simulink model "Task_No5"  (R2023b)
settings: Solver=FixedStepAuto  StartTime=0.0  StopTime=3600*24*7  FixedStep=1  RelTol=1e-3
InitFcn:
  | PARAMETERS;
StartFcn:
  | PARAMETERS;
undefined symbols (not defined in the file): Conv_C_to_K, P_CP_AIR, P_DENSITY_CO2, P_HEATER_AIR_FLOW, P_INIT_CO2, P_M_AIR, P_M_AIR_FLOW, R_WALL, R_WINDOW, RH_INIT_BDR, T_COOLER, T_HEATER, T_INIT_BDR, T_INIT_OUT, TBL_CO2, TBL_TEMP
libraries: fl_lib x32, nesl_utility x20, slpidlib x2
settings Model: Creator=Selim  LastModifiedBy=Selim

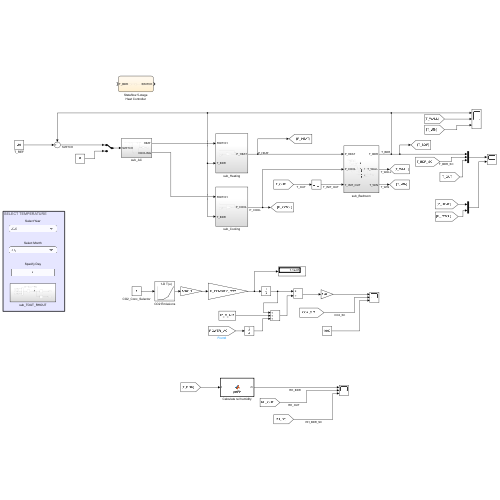
[thumbnail: Simulink's stored preview of the top-level diagram]
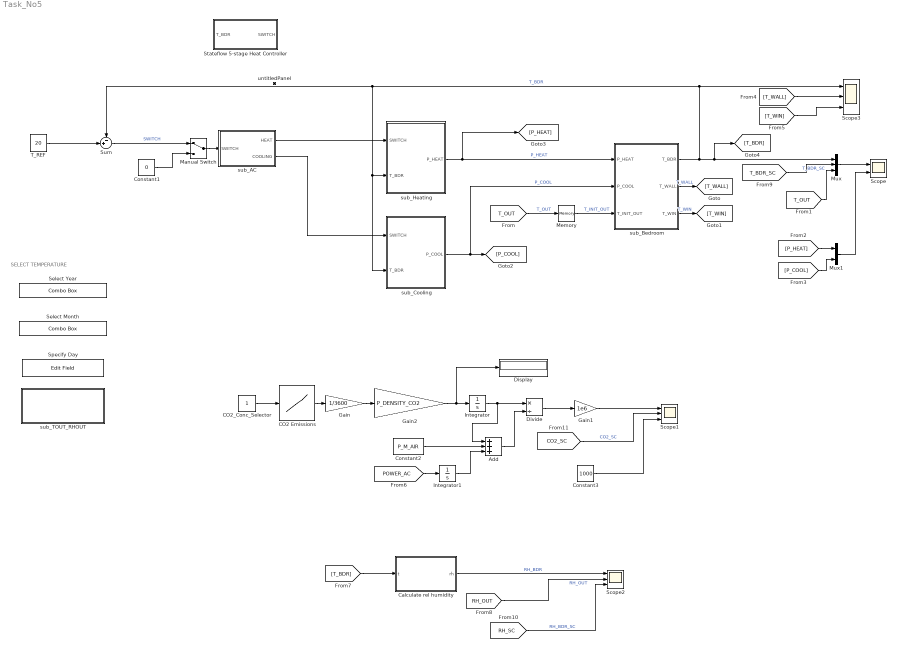
== system Task_No5 ==
  note: SELECT TEMPERATURE
  Add : Sum  Inputs=+++
  CO2 Emissions : Lookup_n-D  NumberOfTableDimensions=1  BreakpointsForDimension1=TBL_CO2.Activity_ID  Table=TBL_CO2.CO2_Emiss_cmh  InternalRulePriority=Speed  RndMeth=Simplest
  CO2_Conc_Selector : Constant
  Calculate rel humidity : MATLAB Function  TreatAsAtomicUnit=on
  Constant1 : Constant  Value=0
  Constant2 : Constant  Value=P_M_AIR
  Constant3 : Constant  Value=1000
  Display : Display
  Divide : Product  Inputs=*/
  Gain : Gain  Gain=1/3600
  Gain1 : Gain  Gain=1e6
  Gain2 : Gain  Gain=P_DENSITY_CO2
  Integrator : Integrator
  Integrator1 : Integrator
  Manual Switch : ManualSwitch
  Memory : Memory  InitialCondition=T_INIT_OUT
  Mux : Mux  Inputs=3
  Mux1 : Mux  Inputs=2
  Scope : Scope  NumInputPorts=2
  Scope1 : Scope  NumInputPorts=3
  Scope2 : Scope  NumInputPorts=3
  Scope3 : Scope  NumInputPorts=3
  Select Month : ComboBox  LabelPosition=Hide  SelectedLabel=July
      settings: Values={{'January', 'February', 'March', 'April', 'May', 'June', 'July', 'August', 'September', 'Oktober', 'November', 'December'}, [1 2 3 4 5 6 7 8 9 10 11 12]}
  Select Year : ComboBox  LabelPosition=Hide  SelectedLabel=2023
      settings: Values={{'2022', '2023'}, [2022 2023]}
  Specify Day : EditField  LabelPosition=Hide  ShowInitialText=on  Alignment=Center
  Stateflow 5-stage Heat Controller : Stateflow chart  TreatAsAtomicUnit=on
  Sum : Sum  Inputs=-+|
  T_REF : Constant  Value=20
  sub_AC : Subsystem
  sub_Bedroom : Subsystem
  sub_Cooling : Subsystem
  sub_Heating : Subsystem
  sub_TOUT_RHOUT : Subsystem
  untitledPanel : Subsystem  Tag=HiddenForWebPanel  IsWebBlockPanel=on
  wires:
  Memory/1 -> sub_Bedroom/3(T_INIT_OUT)  "T_INIT_OUT"
  sub_Bedroom/1(T_BDR) -> [T_BDR], Mux/1, Sum/1, sub_Cooling/2(T_BDR), sub_Heating/2(T_BDR), Scope3/1  "T_BDR"
  sub_Heating/1(P_HEAT) -> [P_HEAT], sub_Bedroom/1(P_HEAT)  "P_HEAT"
  [T_OUT] -> Memory/1  "T_OUT"
  [T_OUT] -> Mux/3
  Mux/1 -> Scope/1
  T_REF/1 -> Sum/2
  Mux1/1 -> Scope/2
  Sum/1 -> Manual Switch/1  "SWITCH"
  sub_AC/1(HEAT) -> sub_Heating/1(SWITCH)
  Manual Switch/1 -> sub_AC/1(SWITCH)
  Constant1/1 -> Manual Switch/2
  sub_Cooling/1(P_COOL) -> [P_COOL], sub_Bedroom/2(P_COOL)  "P_COOL"
  sub_Bedroom/2(T_WALL) -> [T_WALL]  "T_WALL"
  sub_Bedroom/3(T_WIN) -> [T_WIN]  "T_WIN"
  [P_HEAT] -> Mux1/1
  [P_COOL] -> Mux1/2
  [T_WALL] -> Scope3/2
  [T_WIN] -> Scope3/3
  CO2_Conc_Selector/1 -> CO2 Emissions/1
  CO2 Emissions/1 -> Gain/1
  Integrator/1 -> Add/1, Divide/1
  Add/1 -> Divide/2
  Divide/1 -> Gain1/1
  Constant3/1 -> Scope1/3
  Gain1/1 -> Scope1/1
  Gain/1 -> Gain2/1
  Gain2/1 -> Integrator/1, Display/1
  Constant2/1 -> Add/2
  sub_AC/2(COOLING) -> sub_Cooling/1(SWITCH)
  Integrator1/1 -> Add/3
  [POWER_AC] -> Integrator1/1
  Calculate rel humidity/1(rh) -> Scope2/1  "RH_BDR"
  [T_BDR] -> Calculate rel humidity/1(t)
  [RH_OUT] -> Scope2/2  "RH_OUT"
  [T_BDR_SC] -> Mux/2  "T_BDR_SC"
  [RH_SC] -> Scope2/3  "RH_BDR_SC"
  [CO2_SC] -> Scope1/2  "CO2_SC"

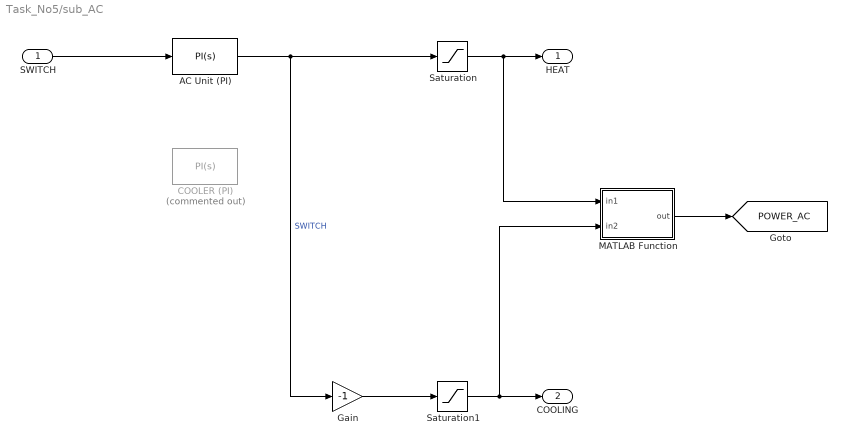
== system Task_No5/sub_AC ==
  SWITCH : Inport
  AC Unit (PI) : slpidlib/PID Controller  Controller=PI  Form=Parallel  TimeDomain=Continuous-time  UseExternalTs=off  SampleTime=-1  IntegratorMethod=Forward Euler  FilterMethod=Forward Euler  ControllerParametersSource=internal  P=0.143081964564318  I=0.00336579194559755  UseKiTs=off  D=39.5738922859411  N=3204.37920267902  UseFilter=on  TunerSelectOption=Transfer Function Based (PID Tuner App)  InitialConditionSource=internal  InitialConditionForIntegrator=0  InitialConditionForFilter=0  DifferentiatorICPrevScaledInput=0  ExternalReset=none  TrackingMode=off  Kt=1  LimitOutput=on  SatLimitsSource=internal  UpperSaturationLimit=1  LowerSaturationLimit=-1  LinearizeAsGain=on  AntiWindupMode=clamping  Kb=1  LimitIntegrator=off  UpperIntegratorSaturationLimit=inf  LowerIntegratorSaturationLimit=-inf  POutMin=[]  POutMax=[]  IOutMin=[]  IOutMax=[]  DOutMin=[]  DOutMax=[]  NOutMin=[]  NOutMax=[]  SumOutMin=[]  SumOutMax=[]  SaturationOutMin=[]  SaturationOutMax=[]  PParamMin=[]  PParamMax=[]  IParamMin=[]  IParamMax=[]  DParamMin=[]  DParamMax=[]  NParamMin=[]  NParamMax=[]  KbParamMin=[]  KbParamMax=[]  KtParamMin=[]  KtParamMax=[]  KbOutMin=[]  KbOutMax=[]  KtOutMin=[]  KtOutMax=[]  IntegratorOutMin=[]  IntegratorOutMax=[]  FilterOutMin=[]  FilterOutMax=[]  SumI1OutMin=[]  SumI1OutMax=[]  SumI2OutMin=[]  SumI2OutMax=[]  SumI3OutMin=[]  SumI3OutMax=[]  SumI4OutMin=[]  SumI4OutMax=[]  SumDOutMin=[]  SumDOutMax=[]  DifferentiatorOutMin=[]  DifferentiatorOutMax=[]  FilterDiffOutCoefMin=[]  FilterDiffOutCoefMax=[]  ReciprocalOutMin=[]  ReciprocalOutMax=[]  SumDenOutMin=[]  SumDenOutMax=[]  SumNumOutMin=[]  SumNumOutMax=[]  DivideOutMin=[]  DivideOutMax=[]  UdiffTsProdOutMin=[]  UdiffTsProdOutMax=[]  NTsProdOutMin=[]  NTsProdOutMax=[]  UintegralTsProdOutMin=[]  UintegralTsProdOutMax=[]  UngainTsProdOutMin=[]  UngainTsProdOutMax=[]  ClampingZeroOutDataTypeStr=Inherit: Inherit via back propagation  ClampingZeroOutMin=[]  ClampingZeroOutMax=[]  FilterDenConstantOutDataTypeStr=Inherit: Inherit via back propagation  FilterDenConstantOutMin=[]  FilterDenConstantOutMax=[]  PCopyOutDataTypeStr=Inherit: Inherit via back propagation  PCopyOutMin=[]  PCopyOutMax=[]  NCopyOutDataTypeStr=Inherit: Inherit via back propagation  NCopyOutMin=[]  NCopyOutMax=[]  IntegratorContinuousStateAttributes=''  IntegratorStateMustResolveToSignalObject=off  IntegratorRTWStateStorageClass=Auto  FilterContinuousStateAttributes=''  FilterStateMustResolveToSignalObject=off  FilterRTWStateStorageClass=Auto  ParallelPVariant=InternalParameters  IdealPVariant=Disabled  IVariant=InternalParameters  DVariant=Disabled  IntegratorVariant=Continuous  SatVariant=Enabled  AWVariant=ContClampingParallel  PCopyVariant=Disabled  TRVariant=Disabled  FdbkBlocksVariant=Forward  IdealPFdbkVariant=Disabled  SatFdbkVariant=Disabled  DerivativeFilterVariant=Disabled  NVariant=Disabled  NCopyVariant=Disabled_SignalSpec  FilterICVariant=Disabled  IntegratorICVariant=InternalICs  ExternalResetVariant=Disabled  TRSumVariant=Passthrough  SumFdbkVariant=Disabled  SumVariant=Sum_PI  TsampFilterVariant=InternalTs  TsampNgainVariant=Passthrough  TsampIntegralVariant=Disabled_SignalSpec  ExternalSaturationOutDataTypeStr=Inherit: Same as second input
  COOLER (PI) : slpidlib/PID Controller  Commented=on  Controller=PI  Form=Parallel  TimeDomain=Continuous-time  UseExternalTs=off  SampleTime=-1  IntegratorMethod=Forward Euler  FilterMethod=Forward Euler  ControllerParametersSource=internal  P=-11.3717981967825  I=-1.40195244638754  UseKiTs=off  D=0  N=100  UseFilter=on  TunerSelectOption=Transfer Function Based (PID Tuner App)  InitialConditionSource=internal  InitialConditionForIntegrator=0  InitialConditionForFilter=0  DifferentiatorICPrevScaledInput=0  ExternalReset=none  TrackingMode=off  Kt=1  LimitOutput=on  SatLimitsSource=internal  UpperSaturationLimit=1  LowerSaturationLimit=0  LinearizeAsGain=on  AntiWindupMode=clamping  Kb=1  LimitIntegrator=off  UpperIntegratorSaturationLimit=inf  LowerIntegratorSaturationLimit=-inf  POutMin=[]  POutMax=[]  IOutMin=[]  IOutMax=[]  DOutMin=[]  DOutMax=[]  NOutMin=[]  NOutMax=[]  SumOutMin=[]  SumOutMax=[]  SaturationOutMin=[]  SaturationOutMax=[]  PParamMin=[]  PParamMax=[]  IParamMin=[]  IParamMax=[]  DParamMin=[]  DParamMax=[]  NParamMin=[]  NParamMax=[]  KbParamMin=[]  KbParamMax=[]  KtParamMin=[]  KtParamMax=[]  KbOutMin=[]  KbOutMax=[]  KtOutMin=[]  KtOutMax=[]  IntegratorOutMin=[]  IntegratorOutMax=[]  FilterOutMin=[]  FilterOutMax=[]  SumI1OutMin=[]  SumI1OutMax=[]  SumI2OutMin=[]  SumI2OutMax=[]  SumI3OutMin=[]  SumI3OutMax=[]  SumI4OutMin=[]  SumI4OutMax=[]  SumDOutMin=[]  SumDOutMax=[]  DifferentiatorOutMin=[]  DifferentiatorOutMax=[]  FilterDiffOutCoefMin=[]  FilterDiffOutCoefMax=[]  ReciprocalOutMin=[]  ReciprocalOutMax=[]  SumDenOutMin=[]  SumDenOutMax=[]  SumNumOutMin=[]  SumNumOutMax=[]  DivideOutMin=[]  DivideOutMax=[]  UdiffTsProdOutMin=[]  UdiffTsProdOutMax=[]  NTsProdOutMin=[]  NTsProdOutMax=[]  UintegralTsProdOutMin=[]  UintegralTsProdOutMax=[]  UngainTsProdOutMin=[]  UngainTsProdOutMax=[]  ClampingZeroOutDataTypeStr=Inherit: Inherit via back propagation  ClampingZeroOutMin=[]  ClampingZeroOutMax=[]  FilterDenConstantOutDataTypeStr=Inherit: Inherit via back propagation  FilterDenConstantOutMin=[]  FilterDenConstantOutMax=[]  PCopyOutDataTypeStr=Inherit: Inherit via back propagation  PCopyOutMin=[]  PCopyOutMax=[]  NCopyOutDataTypeStr=Inherit: Inherit via back propagation  NCopyOutMin=[]  NCopyOutMax=[]  IntegratorContinuousStateAttributes=''  IntegratorStateMustResolveToSignalObject=off  IntegratorRTWStateStorageClass=Auto  FilterContinuousStateAttributes=''  FilterStateMustResolveToSignalObject=off  FilterRTWStateStorageClass=Auto  ParallelPVariant=InternalParameters  IdealPVariant=Disabled  IVariant=InternalParameters  DVariant=Disabled  IntegratorVariant=Continuous  SatVariant=Enabled  AWVariant=ContClampingParallel  PCopyVariant=Disabled  TRVariant=Disabled  FdbkBlocksVariant=Forward  IdealPFdbkVariant=Disabled  SatFdbkVariant=Disabled  DerivativeFilterVariant=Disabled  NVariant=Disabled  NCopyVariant=Disabled_SignalSpec  FilterICVariant=Disabled  IntegratorICVariant=InternalICs  ExternalResetVariant=Disabled  TRSumVariant=Passthrough  SumFdbkVariant=Disabled  SumVariant=Sum_PI  TsampFilterVariant=InternalTs  TsampNgainVariant=Passthrough  TsampIntegralVariant=Disabled_SignalSpec  ExternalSaturationOutDataTypeStr=Inherit: Same as second input
  Gain : Gain  Gain=-1
  MATLAB Function : MATLAB Function  TreatAsAtomicUnit=on
  Saturation : Saturate  UpperLimit=1  LowerLimit=0
  Saturation1 : Saturate  UpperLimit=1  LowerLimit=0
  HEAT : Outport
  COOLING : Outport  Port=2
  tag scope: POWER_AC=global
  wires:
  Gain/1 -> Saturation1/1
  Saturation1/1 -> MATLAB Function/2(in2), COOLING/1
  AC Unit (PI)/1 -> Gain/1, Saturation/1  "SWITCH"
  Saturation/1 -> MATLAB Function/1(in1), HEAT/1
  SWITCH/1 -> AC Unit (PI)/1
  MATLAB Function/1(out) -> [POWER_AC]

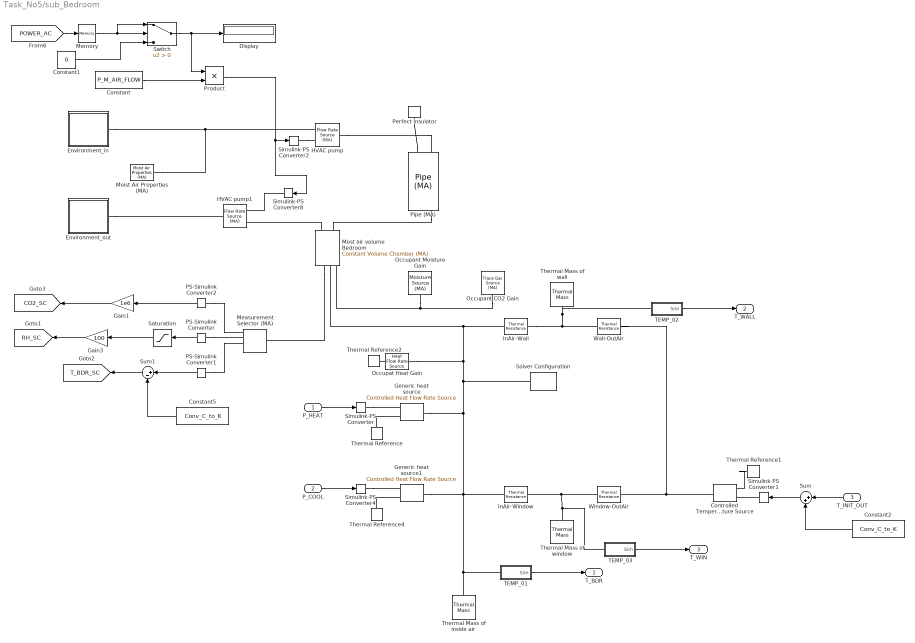
== system Task_No5/sub_Bedroom ==
  P_HEAT : Inport
  P_COOL : Inport  Port=2
  T_INIT_OUT : Inport  Port=3
  Constant : Constant  Value=P_M_AIR_FLOW
  Constant1 : Constant  Value=0
  Constant2 : Constant  Value=Conv_C_to_K
  Constant5 : Constant  Value=Conv_C_to_K
  Controlled Temperature Source : fl_lib/Thermal/Thermal Sources/Controlled Temperature Source
  Display : Display
  Environment_in : Subsystem
  Environment_out : Subsystem
  Gain1 : Gain  Gain=1e6
  Gain3 : Gain  Gain=100
  Generic heat source : fl_lib/Thermal/Thermal Sources/Controlled Heat Flow Rate Source
  Generic heat source1 : fl_lib/Thermal/Thermal Sources/Controlled Heat Flow Rate Source
  HVAC pump : fl_lib/Moist Air/Sources/Flow Rate Source (MA)  source_type=foundation.enum.constant_controlled.controlled  flow_type=foundation.enum.mass_volumetric_flow.mass  mass_flow=0 kg/s  volumetric_flow=0 m^3/s  volumetric_flow_conditions=foundation.enum.volumetric_flow_conditions.actual  p_std=0.101325 MPa  T_std=20 degC  RH_std=0.65  power_spec=foundation.enum.power_spec.isentropic  area_A=P_AREA_DUCT m^2  area_B=P_AREA_DUCT m^2
      settings: InternalSimscapePortConfiguration="{\"Bottom\":[],\"Left\":[{\"id\":\"A\",\"label\":\"A\",\"type\":\"foundation.moist_air.moist_air\"},{\"id\":\"M\",\"label\":\"M\",\"type\":\"input\"}],\"Right\":[{\"id\":\"B\",\"label\":\"B\",\"type\":\"foundation.moist_air.moist_air\"}],\"Top\":[]}"
  HVAC pump1 : fl_lib/Moist Air/Sources/Flow Rate Source (MA)  source_type=foundation.enum.constant_controlled.controlled  flow_type=foundation.enum.mass_volumetric_flow.mass  mass_flow=0 kg/s  volumetric_flow=0 m^3/s  volumetric_flow_conditions=foundation.enum.volumetric_flow_conditions.actual  p_std=0.101325 MPa  T_std=20 degC  RH_std=0.65  power_spec=foundation.enum.power_spec.isentropic  area_A=P_AREA_DUCT m^2  area_B=P_AREA_DUCT m^2
      settings: InternalSimscapePortConfiguration="{\"Bottom\":[],\"Left\":[{\"id\":\"A\",\"label\":\"A\",\"type\":\"foundation.moist_air.moist_air\"},{\"id\":\"M\",\"label\":\"M\",\"type\":\"input\"}],\"Right\":[{\"id\":\"B\",\"label\":\"B\",\"type\":\"foundation.moist_air.moist_air\"}],\"Top\":[]}"
  InAir-Wall : fl_lib/Thermal/Thermal Elements/Thermal Resistance  resistance=R_WALL/2 K/W  T_specify=off  T_priority=None  T=0 K  T_nominal_specify=off  T_nominal_unit=K  T_nominal_value=1  Q_specify=off  Q_priority=None  Q=0 W  Q_nominal_specify=off  Q_nominal_unit=W  Q_nominal_value=1
  InAir-Window : fl_lib/Thermal/Thermal Elements/Thermal Resistance  resistance=R_WINDOW/2 K/W  T_specify=off  T_priority=None  T=0 K  T_nominal_specify=off  T_nominal_unit=K  T_nominal_value=1  Q_specify=off  Q_priority=None  Q=0 W  Q_nominal_specify=off  Q_nominal_unit=W  Q_nominal_value=1
  Measurement Selector (MA) : fl_lib/Moist Air/Sensors/Measurement Selector (MA)  moisture_spec=foundation.enum.moisture_spec.relative_humidity  trace_gas_spec=foundation.enum.trace_gas_spec.mass_fraction
  Memory : Memory
  Moist Air Properties (MA) : fl_lib/Moist Air/Utilities/Moist Air Properties (MA)  R_a=287.047 J/(K*kg)  T_TLU=[-56.55, -50 : 10 : -10, -5 : 1 : 5, 10 : 10 : 350]' degC  h_a_TLU=[342.416126230579; 349.005511058471; 359.063577249119; 369.119948684177; 379.175469465129; 389.230944678417; 394.258910928084; 395.264534937366; 396.27017101329; 397.275819932805; 398.281482472874; 399.287159410541; 400.292851523015; 401.298559587728; 402.304284382408; 403.310026685143; 404.315787274435; 409.34489180313; 419.404921755863; 429.468036401264; 439.535033154839; 449.606720928652; 459.683919949603; 469.767460521911; 479.858181001348; 489.956925196484; 500.064539372946; 510.181869006204; 520.309755403634; 530.449032296018; 540.60052248087; 550.765034584465; 560.943359995745; 571.136270013102; 581.344513234296; 591.568813210327; 601.809866375885; 612.068340261954; 622.344871990218; 632.640067043998; 642.95449830646; 653.288705353699; 663.643193987949; 674.018435994423; 684.414869104228; 694.832897145098; 705.272890361557; 715.735185886199; 726.220088344236; 736.727870574087; 747.258774447567; 757.813011774199] kJ/kg  mu_a_TLU=[14.2568883320012; 14.6140127728333; 15.1517277055779; 15.6806860159119; 16.2012351072083; 16.7137043125028; 16.9670071730589; 17.017438062815; 17.0677930842452; 17.1180725309876; 17.1682766951315; 17.2184058672268; 17.2684603362935; 17.3184403898301; 17.3683463138234; 17.4181783927569; 17.4679369096204; 17.7156358640698; 18.2056751785154; 18.68879035749; 19.1652344664982; 19.6352478927873; 20.099059103658; 20.5568853601578; 21.0089333871663; 21.4554000014051; 21.8964726992323; 22.3323302062775; 22.7631429910631; 23.1890737447833; 23.6102778293792; 24.0269036959922; 24.4390932757886; 24.8469823450548; 25.2507008663546; 25.6503733074314; 26.0461189394339; 26.4380521159325; 26.8262825340948; 27.2109154792923; 27.5920520543128; 27.969789394274; 28.3442208682439; 28.7154362685068; 29.0835219883356; 29.4485611890712; 29.8106339572472; 30.1698174524429; 30.5261860464955; 30.8798114546565; 31.2307628592324; 31.5791070262086] s*uPa  k_a_TLU=[19.8808489374933; 20.4162454629695; 21.2248743590758; 22.0232452890903; 22.8117314495857; 23.5906913619588; 23.9767075412237; 24.053639990175; 24.1304826682191; 24.2072359051629; 24.2839000294007; 24.3604753679152; 24.4369622462801; 24.5133609886625; 24.5896719178249; 24.6658953551279; 24.7420316205333; 25.1214164701832; 25.8738283029331; 26.6180150229276; 27.3542674377332; 28.0828634735341; 28.8040686837224; 29.5181367785657; 30.2253101618423; 30.9258204644224; 31.6198890677835; 32.3077276126633; 32.9895384896798; 33.6655153099498; 34.33584335461; 35.0007000027879; 35.6602551380254; 36.3146715334901; 36.9641052165342; 37.6087058133173; 38.248616874307; 38.8839761815308; 39.5149160384798; 40.1415635435708; 40.7640408480637; 41.3824653993118; 41.9969501701893; 42.6076038755117; 43.2145311762238; 43.8178328720941; 44.4176060836121; 45.013944423749; 45.6069381602018; 46.1966743687041; 46.783237077953; 47.3667074066625] mW/(K*m)  p_min=1 kPa  p_max=inf MPa  T_min=-56.55 degC  T_max=350 degC  properties_range_check=simscape.enum.assert.action.error  p_atm=0.101325 MPa  T_atm=20 degC  R_w=461.523 J/(K*kg)  p_ws_TLU=[1.71168953425982e-06; 3.93770601979424e-06; 1.28411717710344e-05; 3.80051394873809e-05; .00010323902900209; .000259873810798063; .000401741022116384; .000437454836117844; .000476040820618202; .000517704666185737; .000562664883741207; .000611212677444345; .000657088049117899; .000705987905898279; .000758082381149132; .000813549384183233; .000872574861129522; .00122818386934022; .0023392147667769; .00424668834054807; .00738442748706953; .0123512704340234; .0199458019246787; .0312006356960619; .0474147199263783; .0701823607447713; .10141797792131; .143375967241115; .198665399739302; .270259606559999; .361500961984849; .476101381081492; .618139196722055; .792053183687694; 1.0026345688121; 1.25501792086105; 1.55467186826983; 1.90739066433297; 2.31928772772542; 2.79679245576864; 3.34665187151016; 3.97593907083533; 4.69207105435535; 5.5028394740883; 6.41645928168037; 7.4416425436169; 8.58770832955728; 9.86474556030261; 11.2838558865497; 12.8575218898034; 14.6001810568052; 16.5291642526045] MPa  h_w_vap_TLU=[2836.88241275372; 2837.81392500514; 2838.63937175807; 2838.7309929628; 2838.06905313927; 2836.62597341095; 2835.60023952573; 2835.37006381376; 2835.13143158077; 2834.88429145066; 2834.62859062897; 2500.93420564316; 2498.55329907119; 2496.17495082036; 2493.79885912205; 2491.42474723191; 2489.05236104642; 2477.20875029194; 2453.54955988604; 2429.83856603313; 2406.00136954922; 2381.97406342174; 2357.69101156389; 2333.08088387814; 2308.06565480412; 2282.56034405021; 2256.47287422313; 2229.70428017508; 2202.14968030993; 2173.69998896199; 2144.24368406447; 2113.66758247452; 2081.85585110571; 2048.68725710494; 2014.03141249899; 1977.7449923284; 1939.66849592886; 1899.62342931686; 1857.40930169838; 1812.79975416601; 1765.53721731251; 1715.32525772152; 1661.81700477787; 1604.59703745016; 1543.1534616334; 1476.83692476464; 1404.80240352424; 1325.92091736114; 1238.61667822208; 1140.5102987018; 1027.62017777647; 892.733785613825] kJ/kg  h_w_TLU=[2396.55944251649; 2408.68643343608; 2427.1988031141; 2445.702165897; 2464.18429108356; 2482.62529466839; 2491.82135326629; 2493.6580151792; 2495.49372578218; 2497.32843835745; 2499.16210446923; 2500.99462758899; 2502.83092214066; 2504.6665223621; 2506.50140563013; 2508.335548891; 2510.16892865793; 2519.32352241995; 2537.56068088674; 2555.67742615292; 2573.6403223998; 2591.4109179101; 2608.9455037701; 2626.19492016262; 2643.10444358428; 2659.61377634497; 2675.58278696023; 2696.1846256545; 2716.49989553741; 2736.6235210957; 2756.61216047011; 2776.50561773853; 2796.33378922508; 2816.11979583049; 2835.88181423877; 2855.63430574511; 2875.38889327595; 2895.15500577172; 2914.94035964689; 2934.75132290228; 2954.59319330244; 2974.47041285505; 2994.38673458964; 3014.34535328009; 3034.34900867103; 3054.40006755764; 3074.50058946898; 3094.65237953784; 3114.85703128106; 3135.11596137801; 3155.43043805905; 3175.80160435813] kJ/kg  mu_w_TLU=[6.81365662228272; 7.04953750742707; 7.40970098298307; 7.76991278093907; 8.13017290129507; 8.49048134405107; 8.67065368632907; 8.70668960445667; 8.74272600580827; 8.77876289038387; 8.81480025818347; 8.85083810920707; 8.88687644345467; 8.92291526092627; 8.95895456162187; 8.99499434554147; 9.03103461268507; 9.21124319676307; 9.57169660671907; 9.93219833907507; 10.2927483938311; 10.6533467709871; 11.0139934705431; 11.3746884924991; 11.7354318368551; 12.0962235036111; 12.4570634927671; 12.8179518043231; 13.1788884382791; 13.5398733946351; 13.9009066733911; 14.2619882745471; 14.6231181981031; 14.9842964440591; 15.3455230124151; 15.7067979031711; 16.0681211163271; 16.4294926518831; 16.7909125098391; 17.1523806901951; 17.5138971929511; 17.8754620181071; 18.2370751656631; 18.5987366356191; 18.9604464279751; 19.3222045427311; 19.6840109798871; 20.0458657394431; 20.4077688213991; 20.7697202257551; 21.1317199525111; 21.4937680016671] s*uPa  k_w_TLU=[11.46288215976; 11.941997488935; 12.676358586935; 13.414208884935; 14.155548382935; 14.900377080935; 15.274099879935; 15.348949115735; 15.423833243535; 15.498752263335; 15.573706175135; 15.648694978935; 15.723718674735; 15.798777262535; 15.873870742335; 15.948999114135; 16.024162377935; 16.400502076935; 17.155798374935; 17.914583872935; 18.676858570935; 19.442622468935; 20.211875566935; 20.984617864935; 21.760849362935; 22.540570060935; 23.323779958935; 24.110479056935; 24.900667354935; 25.694344852935; 26.491511550935; 27.292167448935; 28.096312546935; 28.903946844935; 29.715070342935; 30.529683040935; 31.347784938935; 32.169376036935; 32.994456334935; 33.823025832935; 34.655084530935; 35.490632428935; 36.329669526935; 37.172195824935; 38.018211322935; 38.867716020935; 39.720709918935; 40.577193016935; 41.437165314935; 42.300626812935; 43.167577510935; 44.038017408935] mW/(K*m)  D_w=25 mm^2/s  trace_gas_model=foundation.enum.trace_gas_model.track_fraction  R_g=188.923 J/(K*kg)  h_g_TLU=[439.555216260064; 444.670268200251; 452.538618847003; 460.487124258496; 468.522588768941; 476.649415958793; 480.74798538725; 481.57054318762; 482.394052398751; 483.218514288831; 484.043930029015; 484.870300696555; 485.697627277859; 486.525910671489; 487.355151691079; 488.185351068185; 489.016509455051; 493.186704139431; 501.599194953048; 510.107689961685; 518.711611080182; 527.410026793075; 536.201764778798; 545.085474203452; 554.059675505208; 563.122805485367; 572.27325096919; 581.509373027928; 590.829525105886; 600.232066705818; 609.715373581392; 619.277845178105; 628.917909922924; 638.634028838794; 648.424697859328; 658.288449140109; 668.223851601449; 678.229510889093; 688.304068901113; 698.44620299875; 708.654624994591; 718.928079991818; 729.265345132425; 739.665228299475; 750.126566808087; 760.648226111439; 771.229098541268; 781.868102096908; 792.564179292476; 803.316296068366; 814.123440770426; 824.984623198037] kJ/kg  mu_g_TLU=[10.8921054191698; 11.2215357085649; 11.7233300740382; 12.2234238147811; 12.7215124453467; 13.2173328890673; 13.4643203184773; 13.5136406274989; 13.562934752385; 13.6122025024997; 13.6614436900741; 13.7106581301692; 13.7598456406398; 13.8090060420983; 13.8581391578796; 13.9072448140062; 13.9563228391538; 14.2012926853717; 14.6890687376044; 15.1738428124161; 15.6554929043332; 16.1339159800463; 16.6090257998657; 17.0807510097148; 17.5490334645512; 18.0138267508952; 18.4750948814453; 18.9328111390399; 19.3869570507278; 19.8375214755778; 20.2844997922255; 20.7278931741254; 21.1677079421287; 21.6039549853963; 22.036649242835; 22.4658092382469; 22.8914566632375; 23.3136160026627; 23.7323141980278; 24.1475803447965; 24.5594454200432; 24.9679420372927; 25.3731042257492; 25.774967231431; 26.1735673380029; 26.5689417053362; 26.9611282240413; 27.350165384404; 27.73609215832; 28.118947892972; 28.4987722151178; 28.8756049449796] s*uPa  k_g_TLU=[10.489430678843; 10.9507672150864; 11.666197960308; 12.392559739764; 13.1299519771612; 13.8778409888416; 14.2554325416312; 14.3312274189707; 14.4071122346908; 14.4830860227061; 14.5591478179508; 14.6352966574703; 14.7115315815553; 14.787851634907; 14.8642558678259; 14.9407433374142; 15.0173131087819; 15.401364480906; 16.1751373988038; 16.9558134611595; 17.7432208682398; 18.5366976599676; 19.3360988502003; 20.1412225692689; 20.9517507672929; 21.7672310558863; 22.5871115634685; 23.4107980865695; 24.2377021890869; 25.0672663781241; 25.8989689893876; 26.732318357514; 27.5668446164644; 28.4020933015927; 29.2376215872816; 30.0729965057542; 30.9077942826816; 31.7416001931033; 32.5740086297993; 33.4046232539953; 34.2330571812868; 35.0589331874899; 35.8818839295189; 36.701552179391; 37.5175910702657; 38.3296643536716; 39.1374466671854; 39.9406238119064; 40.7388930391313; 41.5319633456945; 42.3195557774861; 43.1014037407076] mW/(K*m)  D_g=16 mm^2/s
  Most air volume Bedroom : fl_lib/Moist Air/Elements/Constant Volume Chamber (MA)  volume=P_V_BDR m^3  num_ports=foundation.enum.num_ports.two  area_A=P_AREA_DUCT m^2  area_B=P_AREA_DUCT m^2  area_C=0.01 m^2  area_D=0.01 m^2  RH_ws=1  time_constant=1 s  moisture_trace_gas_source=foundation.enum.moisture_trace_gas_source.controlled  moisture_source_spec=foundation.enum.moisture_source_spec.vapor  moisture_mass_flow=0 kg/s  moisture_temperature_spec=foundation.enum.temperature_spec.atmospheric  moisture_temperature=293.15 K  trace_gas_mass_flow=0 kg/s  trace_gas_temperature_spec=foundation.enum.temperature_spec.atmospheric  trace_gas_temperature=293.15 K  p_I_specify=on  p_I_priority=High  p_I=0.101325 MPa  p_I_nominal_specify=off  p_I_nominal_unit=MPa  p_I_nominal_value=1  T_I_specify=on  T_I_priority=High  T_I=T_INIT_BDR degC  T_I_nominal_specify=off  T_I_nominal_unit=K  T_I_nominal_value=1  RH_I_specify=on  RH_I_priority=High  RH_I=RH_INIT_BDR/100  RH_I_nominal_specify=off  RH_I_nominal_unit=1  RH_I_nominal_value=1  x_w_I_specify=off  x_w_I_priority=None  x_w_I=0  x_w_I_nominal_specify=off  x_w_I_nominal_unit=1  x_w_I_nominal_value=1  y_w_I_specify=off  y_w_I_priority=None  y_w_I=0  y_w_I_nominal_specify=off  y_w_I_nominal_unit=1  y_w_I_nominal_value=1  HR_I_specify=off  HR_I_priority=None  HR_I=0  HR_I_nominal_specify=off  HR_I_nominal_unit=1  HR_I_nominal_value=1  x_g_I_specify=on  x_g_I_priority=High  x_g_I=P_INIT_CO2/1e6  x_g_I_nominal_specify=off  x_g_I_nominal_unit=1  x_g_I_nominal_value=1  y_g_I_specify=off  y_g_I_priority=None  y_g_I=0  y_g_I_nominal_specify=off  y_g_I_nominal_unit=1  y_g_I_nominal_value=1
      settings: InternalSimscapePortConfiguration="{\"Bottom\":[],\"Left\":[{\"id\":\"A\",\"label\":\"A\",\"type\":\"foundation.moist_air.moist_air\"},{\"id\":\"B\",\"label\":\"B\",\"type\":\"foundation.moist_air.moist_air\"}],\"Right\":[{\"id\":\"W\",\"label\":\"W\",\"type\":\"output\"},{\"id\":\"F\",\"label\":\"F\",\"type\":\"output\"},{\"id\":\"H\",\"label\":\"H\",\"type\":\"foundation.thermal.thermal\"},{\"id\":\"S\",\"label\":\"S\",\"type\":\"foundation.moist_air.moist_air_source\"}],\"Top\":[]}"
  Occupant CO2 Gain : fl_lib/Moist Air/Sources/Moisture & Trace Gas Sources/Trace Gas Source (MA)  source_type=foundation.enum.constant_controlled.constant  trace_gas_mass_flow=P_M_HUMAN_CO2 kg/s  temperature_spec=foundation.enum.temperature_spec.specified  trace_gas_temperature=T_BREATH degC  Phi_S_specify=off  Phi_S_priority=None  Phi_S=0 kW  Phi_S_nominal_specify=off  Phi_S_nominal_unit=kW  Phi_S_nominal_value=1  mdot_g_S_specify=off  mdot_g_S_priority=None  mdot_g_S=0 kg/s  mdot_g_S_nominal_specify=off  mdot_g_S_nominal_unit=kg/s  mdot_g_S_nominal_value=1
      settings: InternalSimscapePortConfiguration="{\"Bottom\":[],\"Left\":[{\"id\":\"S\",\"label\":\"S\",\"type\":\"foundation.moist_air.moist_air_source\"}],\"Right\":[],\"Top\":[]}"
  Occupant Moisture Gain : fl_lib/Moist Air/Sources/Moisture & Trace Gas Sources/Moisture Source (MA)  source_type=foundation.enum.constant_controlled.constant  moisture_source_spec=foundation.enum.moisture_source_spec.vapor  moisture_mass_flow=P_M_HUMAN_VAPOR kg/s  temperature_spec=foundation.enum.temperature_spec.specified  moisture_temperature=T_BREATH degC  Phi_S_specify=off  Phi_S_priority=None  Phi_S=0 kW  Phi_S_nominal_specify=off  Phi_S_nominal_unit=kW  Phi_S_nominal_value=1  mdot_w_S_specify=off  mdot_w_S_priority=None  mdot_w_S=0 kg/s  mdot_w_S_nominal_specify=off  mdot_w_S_nominal_unit=kg/s  mdot_w_S_nominal_value=1
      settings: InternalSimscapePortConfiguration="{\"Bottom\":[],\"Left\":[{\"id\":\"S\",\"label\":\"S\",\"type\":\"foundation.moist_air.moist_air_source\"}],\"Right\":[],\"Top\":[]}"
  Occupat Heat Gain : fl_lib/Thermal/Thermal Sources/Heat Flow Rate Source  heat_flow=P_HUMAN W
      settings: InternalSimscapePortConfiguration="{\"Bottom\":[],\"Left\":[{\"id\":\"B\",\"label\":\"B\",\"type\":\"foundation.thermal.thermal\"}],\"Right\":[{\"id\":\"A\",\"label\":\"A\",\"type\":\"foundation.thermal.thermal\"}],\"Top\":[]}"
  PS-Simulink Converter : nesl_utility/PS-Simulink Converter  PhysicalDomain=network_engine_domain  SubClassName=ps_output  LeftPortType=input  RightPortType=output  PseudoPeriodic=off  Frequencies=[]  VectorFormat=inherit  Unit=inherit  AffineConversion=off
  PS-Simulink Converter1 : nesl_utility/PS-Simulink Converter  PhysicalDomain=network_engine_domain  SubClassName=ps_output  LeftPortType=input  RightPortType=output  PseudoPeriodic=off  Frequencies=[]  VectorFormat=inherit  Unit=1  AffineConversion=off
  PS-Simulink Converter2 : nesl_utility/PS-Simulink Converter  PhysicalDomain=network_engine_domain  SubClassName=ps_output  LeftPortType=input  RightPortType=output  PseudoPeriodic=off  Frequencies=[]  VectorFormat=inherit  Unit=inherit  AffineConversion=off
  Perfect Insulator : fl_lib/Thermal/Thermal Elements/Perfect Insulator  T_specify=off  T_priority=None  T=293.15 K  T_nominal_specify=off  T_nominal_unit=K  T_nominal_value=1
  Pipe (MA) : fl_lib/Moist Air/Elements/Pipe (MA)  length=2.5 m  area=P_AREA_DUCT m^2  Dh=P_DIA_DUCT m  length_add=0.1 m  roughness=15e-6 m  Re_lam=2000  Re_tur=4000  shape_factor=64  Nu_lam=3.66  wall_condensation=false  RH_ws=1  time_constant=1e-3 s  moisture_trace_gas_source=foundation.enum.moisture_trace_gas_source.none  moisture_source_spec=foundation.enum.moisture_source_spec.vapor  moisture_mass_flow=0 kg/s  moisture_temperature_spec=foundation.enum.temperature_spec.atmospheric  moisture_temperature=293.15 K  trace_gas_mass_flow=0 kg/s  trace_gas_temperature_spec=foundation.enum.temperature_spec.atmospheric  trace_gas_temperature=293.15 K  p_I_specify=on  p_I_priority=High  p_I=0.101325 MPa  p_I_nominal_specify=off  p_I_nominal_unit=MPa  p_I_nominal_value=1  T_I_specify=on  T_I_priority=High  T_I=T_INIT_BDR degC  T_I_nominal_specify=off  T_I_nominal_unit=K  T_I_nominal_value=1  RH_I_specify=on  RH_I_priority=High  RH_I=RH_INIT_BDR/100  RH_I_nominal_specify=off  RH_I_nominal_unit=1  RH_I_nominal_value=1  x_w_I_specify=off  x_w_I_priority=None  x_w_I=0  x_w_I_nominal_specify=off  x_w_I_nominal_unit=1  x_w_I_nominal_value=1  y_w_I_specify=off  y_w_I_priority=None  y_w_I=0  y_w_I_nominal_specify=off  y_w_I_nominal_unit=1  y_w_I_nominal_value=1  HR_I_specify=off  HR_I_priority=None  HR_I=0  HR_I_nominal_specify=off  HR_I_nominal_unit=1  HR_I_nominal_value=1  x_g_I_specify=on  x_g_I_priority=High  x_g_I=P_INIT_CO2/1e6  x_g_I_nominal_specify=off  x_g_I_nominal_unit=1  x_g_I_nominal_value=1  y_g_I_specify=off  y_g_I_priority=None  y_g_I=0  y_g_I_nominal_specify=off  y_g_I_nominal_unit=1  y_g_I_nominal_value=1
  Product : Product
  Saturation : Saturate  UpperLimit=1  LowerLimit=0
  Simulink-PS Converter{,1..2,4,8} (5 alike) : nesl_utility/Simulink-PS Converter  PhysicalDomain=network_engine_domain  SubClassName=ps_input  LeftPortType=input  RightPortType=output  PseudoPeriodic=off  Frequencies=[]  NoiseDistribution=none  NoiseParameters=[]  Unit=1  AffineConversion=off  FilteringAndDerivatives=provide  SimscapeFilterOrder=1  InputFilterTimeConstant=0.001  UdotUserProvided=0
  Solver Configuration : nesl_utility/Solver Configuration  PhysicalDomain=network_engine_domain  SubClassName=solver  LeftPortType=input  RightPortType=generic  Tones=[]  Harmonics=[]  SimulateNoise=off  Profile=off  UseLocalSampling=off  EnableSwitchedLinearOptims=on  FrequencyDomain=off  UseCCode=off  RelTol=0.001  AbsTol=0.001  MinStep=1e-09  ToWorkspace=off  RevertToSquareIcSolve=off  NumHomotopyIterations=100  PhasorMode=off  PhasorModeNumHarmonics=1  ConsistencySolver=NEWTON_XTOL_AFTER_FTOL  IndexReductionMethod=DerivativeReplacement  DoDC=off  ResidualTolerance=1e-09  ConsistencyTolSource=GLOBAL  ConsistencyAbsTol=0.001  ConsistencyRelTol=0.001  ConsistencyTolFactor=0.001  UseLocalSolver=on  LocalSolverChoice=NE_BACKWARD_EULER_ADVANCER  ResolveIndetEquations=on  FunctionEvalNumThread=1  LocalSolverSampleTime=1  DoFixedCost=on  MaxNonlinIter=3  MaxModeIter=2  ComputeImpulses=off  ImpulseIterations=2  LinearAlgebra=auto  LinearAlgebraNumThread=0  EquationFormulation=NE_TIME_EF  DelaysMemoryBudget=1024  AutomaticFiltering=on  FilteringTimeConstant=0.001  PartitionStorageMethod=AS_NEEDED  PartitionMemoryBudget=1024  PartitionMethod=ROBUST  MultibodyUseLocalSolver=off  MultibodyLocalSolverChoice=ODE1  MultibodyLocalSolverSampleTime=0.001
  Sum : Sum  Inputs=|++
  Sum1 : Sum  Inputs=|+-
  Switch : Switch  Criteria=u2 > Threshold  SaturateOnIntegerOverflow=off  InputSameDT=off
  TEMP_01 : Subsystem
  TEMP_02 : Subsystem
  TEMP_03 : Subsystem
  Thermal Mass of inside air : fl_lib/Thermal/Thermal Elements/Thermal Mass  mass_type=foundation.enum.constant_variable.constant  mass=P_M_AIR kg  sp_heat=P_CP_AIR J/(K*kg)  mass_min=1e-6 kg  num_ports=foundation.enum.numPorts2.one  m_specify=off  m_priority=High  m=1 kg  m_nominal_specify=off  m_nominal_unit=kg  m_nominal_value=1  T_specify=on  T_priority=High  T=T_INIT_BDR degC  T_nominal_specify=off  T_nominal_unit=K  T_nominal_value=1  Q_specify=off  Q_priority=None  Q=0 W  Q_nominal_specify=off  Q_nominal_unit=W  Q_nominal_value=1
  Thermal Mass of wall : fl_lib/Thermal/Thermal Elements/Thermal Mass  mass_type=foundation.enum.constant_variable.constant  mass=P_M_WALL kg  sp_heat=P_CP_WALL J/(K*kg)  mass_min=1e-6 kg  num_ports=foundation.enum.numPorts2.one  m_specify=off  m_priority=High  m=1 kg  m_nominal_specify=off  m_nominal_unit=kg  m_nominal_value=1  T_specify=on  T_priority=High  T=T_INIT_BDR degC  T_nominal_specify=off  T_nominal_unit=K  T_nominal_value=1  Q_specify=off  Q_priority=None  Q=0 W  Q_nominal_specify=off  Q_nominal_unit=W  Q_nominal_value=1
  Thermal Mass of window : fl_lib/Thermal/Thermal Elements/Thermal Mass  mass_type=foundation.enum.constant_variable.constant  mass=P_M_WINDOW kg  sp_heat=P_CP_GLASS J/(K*kg)  mass_min=1e-6 kg  num_ports=foundation.enum.numPorts2.one  m_specify=off  m_priority=High  m=1 kg  m_nominal_specify=off  m_nominal_unit=kg  m_nominal_value=1  T_specify=on  T_priority=High  T=T_INIT_BDR degC  T_nominal_specify=off  T_nominal_unit=K  T_nominal_value=1  Q_specify=off  Q_priority=None  Q=0 W  Q_nominal_specify=off  Q_nominal_unit=W  Q_nominal_value=1
  Thermal Reference{,1..2,4} (4 alike) : fl_lib/Thermal/Thermal Elements/Thermal Reference
  Wall-OutAir : fl_lib/Thermal/Thermal Elements/Thermal Resistance  resistance=R_WINDOW/2 K/W  T_specify=off  T_priority=None  T=0 K  T_nominal_specify=off  T_nominal_unit=K  T_nominal_value=1  Q_specify=off  Q_priority=None  Q=0 W  Q_nominal_specify=off  Q_nominal_unit=W  Q_nominal_value=1
  Window-OutAir : fl_lib/Thermal/Thermal Elements/Thermal Resistance  resistance=R_WINDOW/2 K/W  T_specify=off  T_priority=None  T=0 K  T_nominal_specify=off  T_nominal_unit=K  T_nominal_value=1  Q_specify=off  Q_priority=None  Q=0 W  Q_nominal_specify=off  Q_nominal_unit=W  Q_nominal_value=1
  T_BDR : Outport
  T_WALL : Outport  Port=2
  T_WIN : Outport  Port=3
  tag scope: CO2_SC=global, RH_SC=global, T_BDR_SC=global
  wires:
  Constant2/1 -> Sum/2
  Sum/1 -> Simulink-PS Converter1/1
  TEMP_01/1(Sim) -> T_BDR/1
  P_HEAT/1 -> Simulink-PS Converter/1
  T_INIT_OUT/1 -> Sum/1
  TEMP_02/1(Sim) -> T_WALL/1
  TEMP_03/1(Sim) -> T_WIN/1
  P_COOL/1 -> Simulink-PS Converter4/1
  Constant/1 -> Product/2
  PS-Simulink Converter/1 -> Saturation/1
  Saturation/1 -> Gain3/1
  PS-Simulink Converter1/1 -> Sum1/1
  PS-Simulink Converter2/1 -> Gain1/1
  Gain1/1 -> [CO2_SC]
  Constant5/1 -> Sum1/2
  Sum1/1 -> [T_BDR_SC]
  Gain3/1 -> [RH_SC]
  Product/1 -> Simulink-PS Converter8/1, Simulink-PS Converter2/1
  [POWER_AC] -> Memory/1
  Constant1/1 -> Switch/3
  Switch/1 -> Display/1, Product/1
  Memory/1 -> Switch/1, Switch/2
  connections:
  Thermal Reference/LConn1 -- Generic heat source/RConn2
  Controlled Temperature Source/LConn1 -- Wall-OutAir/RConn1 -- Window-OutAir/RConn1
  Generic heat source/LConn1 -- Solver Configuration/RConn1 -- Most air volume Bedroom/RConn3 -- InAir-Wall/LConn1 -- Occupat Heat Gain/LConn1 -- Generic heat source1/LConn1 -- InAir-Window/LConn1 -- Thermal Mass of inside air/LConn1 -- TEMP_01/LConn1
  Thermal Reference1/LConn1 -- Controlled Temperature Source/RConn2
  Simulink-PS Converter/RConn1 -- Generic heat source/RConn1
  Simulink-PS Converter1/RConn1 -- Controlled Temperature Source/RConn1
  Window-OutAir/LConn1 -- TEMP_03/LConn1 -- Thermal Mass of window/LConn1 -- InAir-Window/RConn1
  InAir-Wall/RConn1 -- TEMP_02/LConn1 -- Thermal Mass of wall/LConn1 -- Wall-OutAir/LConn1
  Simulink-PS Converter4/RConn1 -- Generic heat source1/RConn1
  Thermal Reference4/LConn1 -- Generic heat source1/RConn2
  Thermal Reference2/LConn1 -- Occupat Heat Gain/RConn1
  Occupant Moisture Gain/LConn1 -- Most air volume Bedroom/RConn4 -- Occupant CO2 Gain/LConn1
  HVAC pump/RConn1 -- Pipe (MA)/LConn1
  Simulink-PS Converter2/RConn1 -- HVAC pump/LConn2
  Most air volume Bedroom/RConn2 -- Measurement Selector (MA)/LConn1
  PS-Simulink Converter/LConn1 -- Measurement Selector (MA)/RConn3
  PS-Simulink Converter1/LConn1 -- Measurement Selector (MA)/RConn2
  PS-Simulink Converter2/LConn1 -- Measurement Selector (MA)/RConn4
  Pipe (MA)/RConn1 -- Most air volume Bedroom/LConn2
  Perfect Insulator/LConn1 -- Pipe (MA)/LConn2
  Simulink-PS Converter8/RConn1 -- HVAC pump1/LConn2
  Most air volume Bedroom/LConn1 -- HVAC pump1/LConn1
  Environment_out/LConn1 -- HVAC pump1/RConn1
  Moist Air Properties (MA)/RConn1 -- Environment_in/LConn1 -- HVAC pump/LConn1

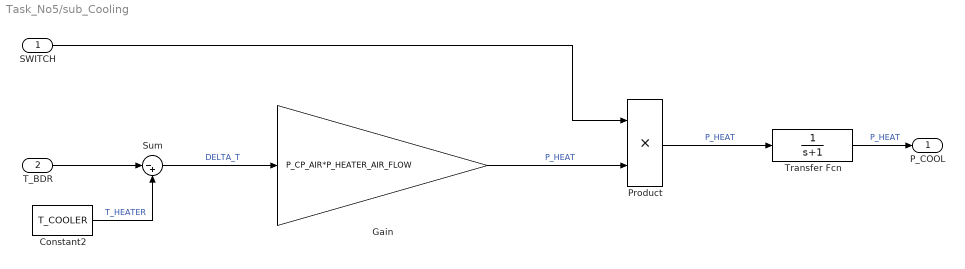
== system Task_No5/sub_Cooling ==
  SWITCH : Inport
  T_BDR : Inport  Port=2
  Constant2 : Constant  Value=T_COOLER
  Gain : Gain  Gain=P_CP_AIR*P_HEATER_AIR_FLOW
  Product : Product
  Sum : Sum  Inputs=|-+
  Transfer Fcn : TransferFcn  Denominator=[1 1]
  P_COOL : Outport
  wires:
  Product/1 -> Transfer Fcn/1  "P_HEAT"
  T_BDR/1 -> Sum/1
  Gain/1 -> Product/2  "P_HEAT"
  SWITCH/1 -> Product/1
  Constant2/1 -> Sum/2  "T_HEATER"
  Transfer Fcn/1 -> P_COOL/1  "P_HEAT"
  Sum/1 -> Gain/1  "DELTA_T"

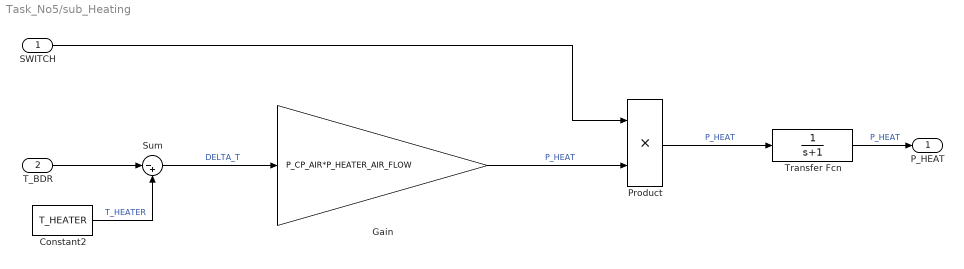
== system Task_No5/sub_Heating ==
  SWITCH : Inport
  T_BDR : Inport  Port=2
  Constant2 : Constant  Value=T_HEATER
  Gain : Gain  Gain=P_CP_AIR*P_HEATER_AIR_FLOW
  Product : Product
  Sum : Sum  Inputs=|-+
  Transfer Fcn : TransferFcn  Denominator=[1 1]
  P_HEAT : Outport
  wires:
  Sum/1 -> Gain/1  "DELTA_T"
  Transfer Fcn/1 -> P_HEAT/1  "P_HEAT"
  Constant2/1 -> Sum/2  "T_HEATER"
  SWITCH/1 -> Product/1
  Gain/1 -> Product/2  "P_HEAT"
  T_BDR/1 -> Sum/1
  Product/1 -> Transfer Fcn/1  "P_HEAT"

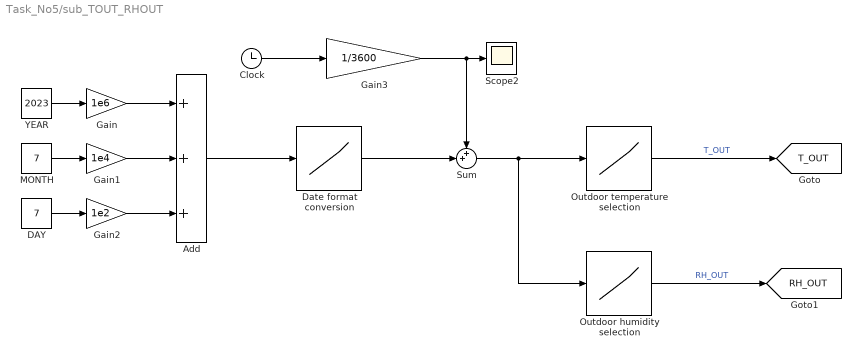
== system Task_No5/sub_TOUT_RHOUT ==
  Add : Sum  Inputs=+++
  Clock : Clock
  DAY : Constant  Value=7
  Date format conversion : Lookup_n-D  NumberOfTableDimensions=1  BreakpointsForDimension1=TBL_TEMP.DATE_yyyymmddhh  Table=TBL_TEMP.DATE_sec  InternalRulePriority=Speed  RndMeth=Simplest
  Gain : Gain  Gain=1e6
  Gain1 : Gain  Gain=1e4
  Gain2 : Gain  Gain=1e2
  Gain3 : Gain  Gain=1/3600
  MONTH : Constant  Value=7
  Outdoor humidity selection : Lookup_n-D  NumberOfTableDimensions=1  BreakpointsForDimension1=TBL_TEMP.DATE_sec  Table=TBL_TEMP.RM_p100  InternalRulePriority=Speed  RndMeth=Simplest
  Outdoor temperature selection : Lookup_n-D  NumberOfTableDimensions=1  BreakpointsForDimension1=TBL_TEMP.DATE_sec  Table=TBL_TEMP.T_C  InternalRulePriority=Speed  RndMeth=Simplest
  Scope2 : Scope
  Sum : Sum  Inputs=++|
  YEAR : Constant  Value=2023
  tag scope: RH_OUT=global, T_OUT=global
  wires:
  Gain1/1 -> Add/2
  MONTH/1 -> Gain1/1
  Clock/1 -> Gain3/1
  Date format conversion/1 -> Sum/2
  Add/1 -> Date format conversion/1
  YEAR/1 -> Gain/1
  Gain/1 -> Add/1
  Gain3/1 -> Scope2/1, Sum/1
  Sum/1 -> Outdoor humidity selection/1, Outdoor temperature selection/1
  Gain2/1 -> Add/3
  DAY/1 -> Gain2/1
  Outdoor temperature selection/1 -> [T_OUT]  "T_OUT"
  Outdoor humidity selection/1 -> [RH_OUT]  "RH_OUT"

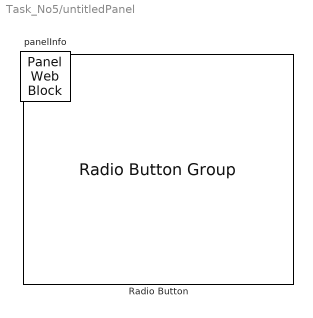
== system Task_No5/untitledPanel ==
  Radio Button : RadioButtonGroup  Tag=HiddenForWebPanel  PanelInfo="{\"addnFilesFolder\":\"\",\"height\":230,\"includeDebugPackages\":false,\"left\":18,\"outputFolder\":\"\",\"panelId\":\"panelId-a10107d6-1e7d-451d-956e-0df6eada92c1\",\"popoutMode\":\"\",\"standaloneTitle\":\"\",\"top\":18,\"type\":\"panelChild\",\"version\":\"2019b\",\"width\":270,\"zIndex\":1500002}"  SelectedLabel=Label3  ButtonGroupName=Group
      settings: Values={{'Label1', 'Label2', 'Label3'}, [0 1 2]}
  panelInfo : PanelWebBlock  Tag=HiddenForWebPanel  PanelInfo="{\"addnFilesFolder\":\"\",\"compacted\":false,\"height\":270,\"includeDebugPackages\":false,\"isActiveTab\":true,\"left\":296,\"name\":\"Panel\",\"outputFolder\":\"\",\"panelId\":\"panelId-a10107d6-1e7d-451d-956e-0df6eada92c1\",\"popoutData\":{\"height\":334,\"left\":361,\"maximized\":false,\"top\":306,\"width\":324},\"popoutMode\":\"windowHidden\",\"standaloneTitle\":\"\",\"tabIndex\":0,\"tabbedSetId\":\"tabbedSet8433950298\",\"top\":135,\"type\":\"panel\",\"version\":\"2019b\",\"visible\":true,\"width\":310,\"zIndex\":1500002}"

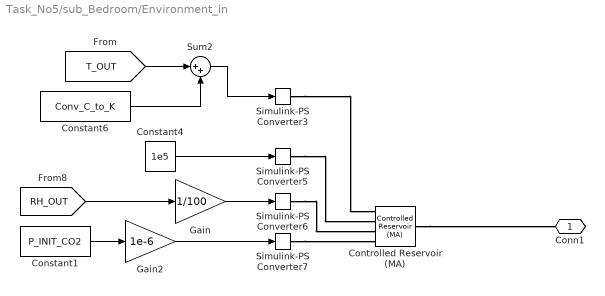
== system Task_No5/sub_Bedroom/Environment_in ==
  Constant1 : Constant  Value=P_INIT_CO2
  Constant4 : Constant  Value=1e5
  Constant6 : Constant  Value=Conv_C_to_K
  Controlled Reservoir (MA) : fl_lib/Moist Air/Elements/Controlled Reservoir (MA)  moisture_spec=foundation.enum.moistureSpec.RelativeHumidity  trace_gas_spec=foundation.enum.trace_gas_spec.mass_fraction  RH_ws=1  area_A=P_AREA_DUCT m^2  input_error_spec=foundation.enum.input_range_error.warn
      settings: InternalSimscapePortConfiguration="{\"Bottom\":[],\"Left\":[{\"id\":\"A\",\"label\":\"A\",\"type\":\"foundation.moist_air.moist_air\"}],\"Right\":[{\"id\":\"T\",\"label\":\"T\",\"type\":\"input\"},{\"id\":\"P\",\"label\":\"P\",\"type\":\"input\"},{\"id\":\"W\",\"label\":\"W\",\"type\":\"input\"},{\"id\":\"G\",\"label\":\"G\",\"type\":\"input\"}],\"Top\":[]}"
  Gain : Gain  Gain=1/100
  Gain2 : Gain  Gain=1e-6
  Simulink-PS Converter{3,5..7} (4 alike) : nesl_utility/Simulink-PS Converter  PhysicalDomain=network_engine_domain  SubClassName=ps_input  LeftPortType=input  RightPortType=output  PseudoPeriodic=off  Frequencies=[]  NoiseDistribution=none  NoiseParameters=[]  Unit=1  AffineConversion=off  FilteringAndDerivatives=provide  SimscapeFilterOrder=1  InputFilterTimeConstant=0.001  UdotUserProvided=0
  Sum2 : Sum  Inputs=|++
  Conn1 : PMIOPort  Side=Left
  wires:
  Constant1/1 -> Gain2/1
  Constant6/1 -> Sum2/2
  Gain/1 -> Simulink-PS Converter6/1
  Constant4/1 -> Simulink-PS Converter5/1
  Gain2/1 -> Simulink-PS Converter7/1
  Sum2/1 -> Simulink-PS Converter3/1
  [T_OUT] -> Sum2/1
  [RH_OUT] -> Gain/1
  connections:
  Simulink-PS Converter3/RConn1 -- Controlled Reservoir (MA)/RConn1
  Simulink-PS Converter7/RConn1 -- Controlled Reservoir (MA)/RConn4
  Controlled Reservoir (MA)/LConn1 -- Conn1/RConn1
  Simulink-PS Converter5/RConn1 -- Controlled Reservoir (MA)/RConn2
  Simulink-PS Converter6/RConn1 -- Controlled Reservoir (MA)/RConn3

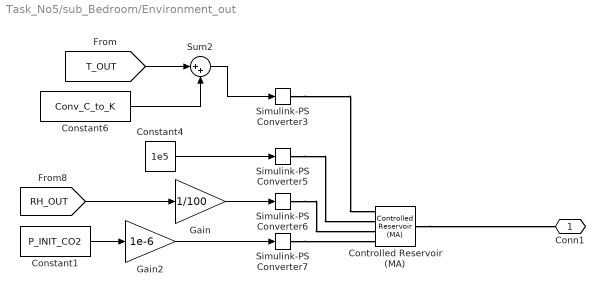
== system Task_No5/sub_Bedroom/Environment_out ==
  Constant1 : Constant  Value=P_INIT_CO2
  Constant4 : Constant  Value=1e5
  Constant6 : Constant  Value=Conv_C_to_K
  Controlled Reservoir (MA) : fl_lib/Moist Air/Elements/Controlled Reservoir (MA)  moisture_spec=foundation.enum.moistureSpec.RelativeHumidity  trace_gas_spec=foundation.enum.trace_gas_spec.mass_fraction  RH_ws=1  area_A=P_AREA_DUCT m^2  input_error_spec=foundation.enum.input_range_error.warn
      settings: InternalSimscapePortConfiguration="{\"Bottom\":[],\"Left\":[{\"id\":\"A\",\"label\":\"A\",\"type\":\"foundation.moist_air.moist_air\"}],\"Right\":[{\"id\":\"T\",\"label\":\"T\",\"type\":\"input\"},{\"id\":\"P\",\"label\":\"P\",\"type\":\"input\"},{\"id\":\"W\",\"label\":\"W\",\"type\":\"input\"},{\"id\":\"G\",\"label\":\"G\",\"type\":\"input\"}],\"Top\":[]}"
  Gain : Gain  Gain=1/100
  Gain2 : Gain  Gain=1e-6
  Simulink-PS Converter{3,5..7} (4 alike) : nesl_utility/Simulink-PS Converter  PhysicalDomain=network_engine_domain  SubClassName=ps_input  LeftPortType=input  RightPortType=output  PseudoPeriodic=off  Frequencies=[]  NoiseDistribution=none  NoiseParameters=[]  Unit=1  AffineConversion=off  FilteringAndDerivatives=provide  SimscapeFilterOrder=1  InputFilterTimeConstant=0.001  UdotUserProvided=0
  Sum2 : Sum  Inputs=|++
  Conn1 : PMIOPort  Side=Left
  wires:
  [RH_OUT] -> Gain/1
  [T_OUT] -> Sum2/1
  Sum2/1 -> Simulink-PS Converter3/1
  Gain2/1 -> Simulink-PS Converter7/1
  Constant4/1 -> Simulink-PS Converter5/1
  Gain/1 -> Simulink-PS Converter6/1
  Constant6/1 -> Sum2/2
  Constant1/1 -> Gain2/1
  connections:
  Simulink-PS Converter6/RConn1 -- Controlled Reservoir (MA)/RConn3
  Simulink-PS Converter5/RConn1 -- Controlled Reservoir (MA)/RConn2
  Controlled Reservoir (MA)/LConn1 -- Conn1/RConn1
  Simulink-PS Converter7/RConn1 -- Controlled Reservoir (MA)/RConn4
  Simulink-PS Converter3/RConn1 -- Controlled Reservoir (MA)/RConn1

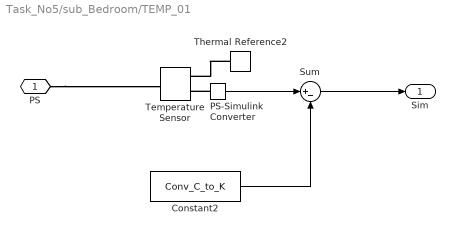
== system Task_No5/sub_Bedroom/TEMP_01 ==
  Constant2 : Constant  Value=Conv_C_to_K
  PS-Simulink Converter : nesl_utility/PS-Simulink Converter  PhysicalDomain=network_engine_domain  SubClassName=ps_output  LeftPortType=input  RightPortType=output  PseudoPeriodic=off  Frequencies=[]  VectorFormat=inherit  Unit=inherit  AffineConversion=off
  Sum : Sum  Inputs=|+-
  Temperature Sensor : fl_lib/Thermal/Thermal Sensors/Temperature Sensor  temperature_measure=foundation.enum.MeasurementReference.difference
  Thermal Reference2 : fl_lib/Thermal/Thermal Elements/Thermal Reference
  PS : PMIOPort  Side=Left
  Sim : Outport
  wires:
  Sum/1 -> Sim/1
  PS-Simulink Converter/1 -> Sum/1
  Constant2/1 -> Sum/2
  connections:
  Thermal Reference2/LConn1 -- Temperature Sensor/RConn1
  PS-Simulink Converter/LConn1 -- Temperature Sensor/RConn2
  PS/RConn1 -- Temperature Sensor/LConn1

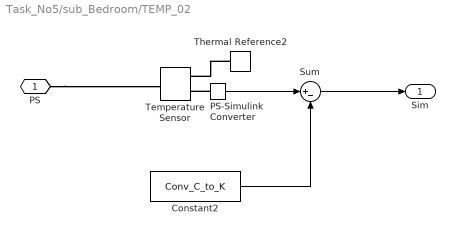
== system Task_No5/sub_Bedroom/TEMP_02 ==
  Constant2 : Constant  Value=Conv_C_to_K
  PS-Simulink Converter : nesl_utility/PS-Simulink Converter  PhysicalDomain=network_engine_domain  SubClassName=ps_output  LeftPortType=input  RightPortType=output  PseudoPeriodic=off  Frequencies=[]  VectorFormat=inherit  Unit=inherit  AffineConversion=off
  Sum : Sum  Inputs=|+-
  Temperature Sensor : fl_lib/Thermal/Thermal Sensors/Temperature Sensor  temperature_measure=foundation.enum.MeasurementReference.difference
  Thermal Reference2 : fl_lib/Thermal/Thermal Elements/Thermal Reference
  PS : PMIOPort  Side=Left
  Sim : Outport
  wires:
  Sum/1 -> Sim/1
  PS-Simulink Converter/1 -> Sum/1
  Constant2/1 -> Sum/2
  connections:
  Thermal Reference2/LConn1 -- Temperature Sensor/RConn1
  PS-Simulink Converter/LConn1 -- Temperature Sensor/RConn2
  PS/RConn1 -- Temperature Sensor/LConn1

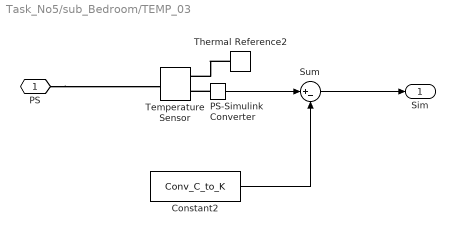
== system Task_No5/sub_Bedroom/TEMP_03 ==
  Constant2 : Constant  Value=Conv_C_to_K
  PS-Simulink Converter : nesl_utility/PS-Simulink Converter  PhysicalDomain=network_engine_domain  SubClassName=ps_output  LeftPortType=input  RightPortType=output  PseudoPeriodic=off  Frequencies=[]  VectorFormat=inherit  Unit=inherit  AffineConversion=off
  Sum : Sum  Inputs=|+-
  Temperature Sensor : fl_lib/Thermal/Thermal Sensors/Temperature Sensor  temperature_measure=foundation.enum.MeasurementReference.difference
  Thermal Reference2 : fl_lib/Thermal/Thermal Elements/Thermal Reference
  PS : PMIOPort  Side=Left
  Sim : Outport
  wires:
  Sum/1 -> Sim/1
  PS-Simulink Converter/1 -> Sum/1
  Constant2/1 -> Sum/2
  connections:
  Thermal Reference2/LConn1 -- Temperature Sensor/RConn1
  PS-Simulink Converter/LConn1 -- Temperature Sensor/RConn2
  PS/RConn1 -- Temperature Sensor/LConn1

== stateflow chart Task_No5/Stateflow 5-stage Heat Controller ==
  state Off
    entry:
    SWITCH = 0;
  state Low
    entry:
    SWITCH = 0.25;
  state Medium
    entry:
    SWITCH = 0.5;
  state High
    entry:
    SWITCH = 0.75;
  state Full
    entry:
    SWITCH = 1;
  (default) -> Off
  Low -> Medium [order 2] : [T_BDR<20]
  High -> Full [order 2] : [T_BDR<18]
  Off -> Low : [T_BDR<21]
  Medium -> High [order 2] : [T_BDR<19]
  Low -> Off [order 1] : [T_BDR>=22]
  Medium -> Low [order 1] : [T_BDR>=21]
  High -> Medium [order 1] : [T_BDR>=20]
  Full -> High : [T_BDR>=20]
  data: T_BDR input; SWITCH output

== matlab function Task_No5/sub_AC/MATLAB Function ==
  data: in1 input; out output; in2 input
function out = fcn(in1, in2)

if in1 == 0 && in2 > 0
    out = in2;
else
    out = in1;
end

== matlab function Task_No5/Calculate rel humidity ==
  data: rh output; t input; RH_INIT_BDR parameter; T_INIT_BDR parameter
function rh = getRH(t, RH_INIT_BDR, T_INIT_BDR)

    es1 = magnus(T_INIT_BDR);
    es2 = magnus(t);
    e1 = RH_INIT_BDR * es1 / 100;

    rh = e1 / es2 * 100;

function es = magnus(t)
    es = 6.112*exp(17.62*t/(243.12+t));
end
end
